simulink model "observer_feedback_model"  (R2023b)
settings: Solver=VariableStepAuto  StartTime=0.0  StopTime=10  RelTol=1e-3
libraries: simulink_extras x3, dspsigattribs x1, cstblocks x1, spspowerguiLib x1
settings Model: Creator=dimia  LastModifiedBy=dimia

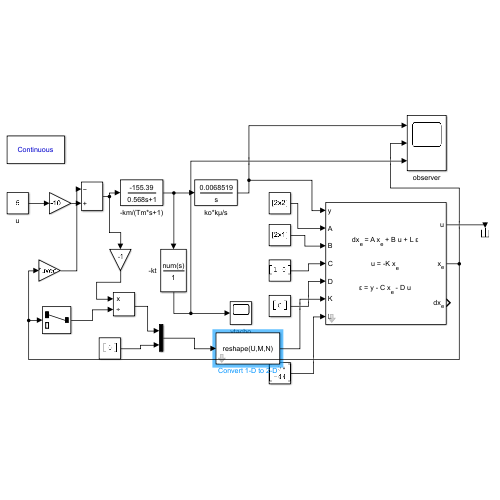
[thumbnail: Simulink's stored preview of the top-level diagram]
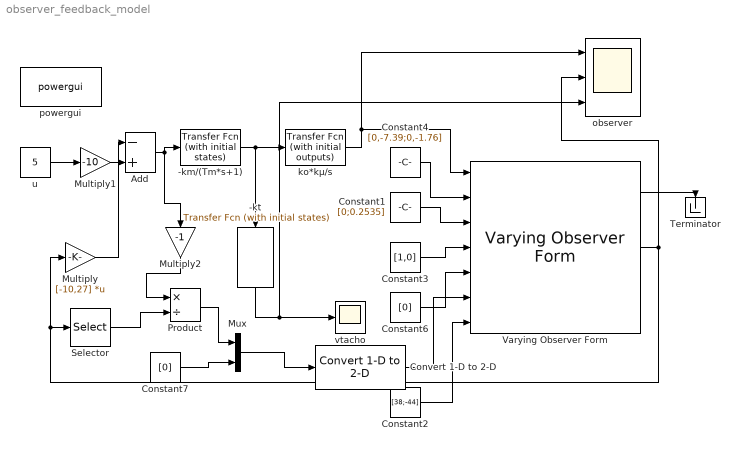
== system observer_feedback_model ==
  -km/(Tm*s+1) : simulink_extras/Additional Linear/Transfer Fcn (with initial states)  N=[-155.39]  D=[0.568 1]  X0=0
  -kt : simulink_extras/Additional Linear/Transfer Fcn (with initial states)  N=-9.2667*10^(-4)  D=[1]  X0=0
  Add : Sum  Inputs=-+
  Constant1 : Constant  Value=[0;0.2535]  VectorParams1D=off
  Constant2 : Constant  Value=[38;-44]  VectorParams1D=off
  Constant3 : Constant  Value=[1,0]  VectorParams1D=off
  Constant4 : Constant  Value=[0,-7.39;0,-1.76]  VectorParams1D=off
  Constant6 : Constant  Value=[0]  VectorParams1D=off
  Constant7 : Constant  Value=[0]  VectorParams1D=off
  Convert 1-D to 2-D : dspsigattribs/Convert 1-D to 2-D  M=1  N=2  frameBasedOut=off
  Multiply : Gain  Gain=[-10,27]  Multiplication=Matrix(K*u) (u vector)
  Multiply1 : Gain  Gain=-10
  Multiply2 : Gain  Gain=-1
  Mux : Mux  Inputs=2
  Product : Product  Inputs=*/
  Selector : Selector  InputPortWidth=2  IndexOptions=Index vector (dialog)  Indices=1  OutputSizes=1
  Terminator : Terminator
  Varying Observer Form : cstblocks/Linear Parameter Varying/Varying Observer Form  x0=[2,0]  xNames=''  OutputX=on  OutputDX=on
  ko*kμ/s : simulink_extras/Additional Linear/Transfer Fcn (with initial outputs)  N=[(1/36)*0.24667]  D="[1  0]"  Y0=2  U0=0
  observer : Scope  NumInputPorts=3
  powergui : spspowerguiLib/powergui  Priority=1  SimulationMode=Continuous  SampleTime=50e-6  frequency=60  Iterations=50  frequencyindice=60  Pbase=100e6  ErrMax=1e-4  UnitsV=kV  UnitsW=MW  buscounter=0  FunctionMessages=off  echomessages=off  EnableUseOfTLC=off  CurrentSourceSwitches=off  DisableSnubberDevices=off  DisableRonSwitches=off  DisableVfSwitches=off  DisplayEquations=off  AutomaticDiscreteSolvers=off  SolverType=Tustin/Backward Euler (TBE)  Interpol=off  ExternalGateDelay=off  methode=off  Ts=100  x0status=blocks  SPID=on  SwTol=0  HookPort=off  NonlinearTolerance=1e-4  nMaxIteration=100  ContinueOnMaxIteration=off  RestoreLinks=warning  ResistiveCurrentMeasurement=off  Frange=[0:2:500]  Ylog=off  Xlog=on  ShowGrid=off  save=off  variable=ZData  structure=0  ZoomFFT=off  StartTime=0.0  cycles=1  DisplayStyle=1  fundamental=60  FreqAxis=off  MaxFrequency=1000  frequencyindicesteady=1  RmsSteady=1  display=off
  u : Constant  Value=5
  vtacho : Scope
  wires:
  Add/1 -> Multiply2/1, -km/(Tm*s+1)/1
  u/1 -> Multiply1/1
  -km/(Tm*s+1)/1 -> ko*kμ/s/1, -kt/1
  Multiply1/1 -> Add/2
  -kt/1 -> vtacho/1, observer/3
  Constant1/1 -> Varying Observer Form/3
  Constant2/1 -> Varying Observer Form/7
  Constant3/1 -> Varying Observer Form/4
  Constant6/1 -> Varying Observer Form/5
  Mux/1 -> Convert 1-D to 2-D/1
  Constant4/1 -> Varying Observer Form/2
  Varying Observer Form/2 -> observer/2, Selector/1, Multiply/1
  ko*kμ/s/1 -> observer/1, Varying Observer Form/1
  Multiply/1 -> Add/1
  Varying Observer Form/1 -> Terminator/1
  Multiply2/1 -> Product/1
  Selector/1 -> Product/2
  Product/1 -> Mux/1
  Constant7/1 -> Mux/2
  Convert 1-D to 2-D/1 -> Varying Observer Form/6
